simulink model "plant_for_linear_analysis"  (R2015a)
settings: Solver=ode45  StartTime=0.0  StopTime=10.0  RelTol=1e-3
undefined symbols (not defined in the file or in its folder): magnitude
settings Model: Creator=Jack  LastModifiedBy=Jack

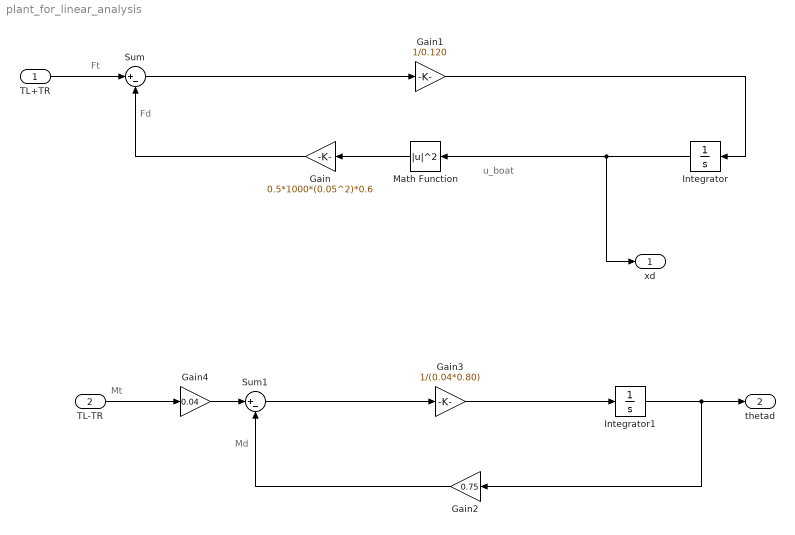
== system plant_for_linear_analysis ==
  note: Ft
  note: Fd
  note: u_boat
  note: Mt
  note: Md
  TL+TR : Inport
  TL-TR : Inport  Port=2
  Gain : Gain  Gain=0.5*1000*(0.05^2)*0.6
  Gain1 : Gain  Gain=1/0.120
  Gain2 : Gain  Gain=0.75
  Gain3 : Gain  Gain=1/(0.04*0.80)
  Gain4 : Gain  Gain=0.04
  Integrator : Integrator  InitialCondition=1.0  ContinuousStateAttributes='u_boat'
  Integrator1 : Integrator  InitialCondition=1.0  ContinuousStateAttributes='theta_d'
  Math Function : Math  Operator=magnitude^2  SaturateOnIntegerOverflow=on
  Sum : Sum  Inputs=|+-
  Sum1 : Sum  Inputs=|+-
  xd : Outport
  thetad : Outport  Port=2
  wires:
  TL+TR/1 -> Sum/1
  Sum/1 -> Gain1/1
  Integrator/1 -> xd/1, Math Function/1
  Gain/1 -> Sum/2
  Gain1/1 -> Integrator/1
  Math Function/1 -> Gain/1
  Sum1/1 -> Gain3/1
  Integrator1/1 -> Gain2/1, thetad/1
  Gain2/1 -> Sum1/2
  Gain3/1 -> Integrator1/1
  Gain4/1 -> Sum1/1
  TL-TR/1 -> Gain4/1
